simulink library "qcatlib"  (R2015a)
settings: Solver=ode45  SolverMode=SingleTasking  StartTime=0.0  StopTime=10.0  RelTol=1e-3
undefined symbols (not defined in the file or in its folder): dyn_ca_sl, qp_ca_sl
settings Model: CovSFcnEnable=off  ExtModeAutoUpdateStatusClock=off  Creator=ola  LastModifiedBy=David
settings DataIOCC: SignalLoggingSaveFormat=ModelDataLogs
settings OptimizationCC: BlockReduction=off  BooleanDataType=off  ExpressionDepthLimit=2147483647
settings DebuggingCC: SaveWithParameterizedLinksMsg=none  UnderspecifiedInitializationDetection=Classic  MergeDetectMultiDrivingBlocksExec=none  SignalResolutionControl=TryResolveAllWithWarning  MultiTaskDSMMsg=warning  MultiTaskCondExecSysMsg=none  StateNameClashWarn=warning  StrictBusMsg=None
settings HardwareCC: TargetUnknown=on

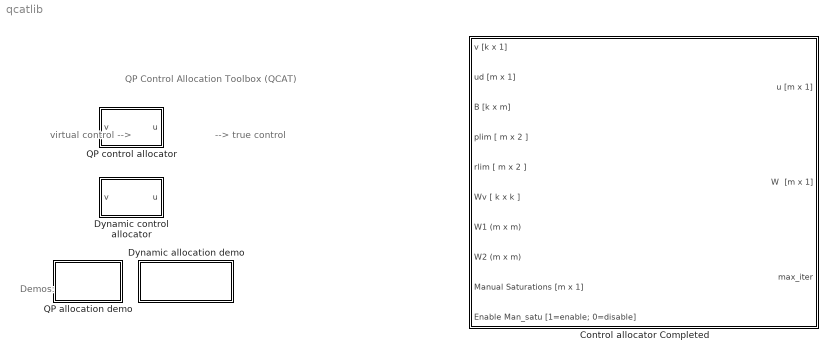
== system qcatlib ==
  note: virtual control -->
  note: --> true control
  note: QP Control Allocation Toolbox (QCAT)
  note: Demos:
  "Control allocator Completed " : Subsystem  TreatAsAtomicUnit=on  mask(Control allocator Completed){alg=WLS, CA_type=DYN, iter_max=100, gamma=1e6, k_B=3, m_B=7, T=0.01, tol=0}
      mask prompts: alg "Algorithm"; CA_type "CA type: Perform Dynamic CA?"; iter_max "Maximum number of iterations"; gamma "Weight of Control Error Cost (gamma) (If SLS, MLS or CGI:Include it in Wv)"; k_B "Number of rows B matrix"; m_B "Number of columns B Matrix"; T "Sample Time"; tol "Tolerance, tol"
      mask help:
      | Author: David Torres
      | Based on work of Ola Härkegård
      |
      | Given the virtual control command v:
      |  The control input u is computed using dynamic control allocation (see help dyn_ca_COMP).
      | OR
      |  The control input u is computed using l2-optimal control allocation (see help qp_ca_COMP).
      |
      | Type qcatdoc for more information.
      |
      | Note: CGI,FXP and IP do not manage saturations.
      mask Help: See the documentation for CA_COMP , dyn_ca_COMP or qp_ca_COMP.
      mask TypeOptions alg: SLS | WLS | WLSC | MLS | IP | CGI | FXP
      mask Callback alg:
      | val = get_param(gcb,'MaskValues');
      | switch lower(val{1})
      |  case {'sls','mls','cgi'}
      |   set_param(gcb,'MaskVisibilities',{'on','on','on','off','on','on','on','off'});
      |  case {'wls','wlsc','fxp'}
      |   set_param(gcb,'MaskVisibilities',{'on','on','on','on','on','on','on','off'});
      |  case {'ip'}
      |   set_param(gcb,'MaskVisibilities',{'on','on','on','on','on','on','on','on'});
      | end
      mask TypeOptions CA_type: DYN | QP
      mask Display:
      | fprintf('%s',upper(alg))
      | % %
      | % %
      | % % port_label('output', 1, 'u [m x 1]')
      | % % port_label('output', 2, 'W [m x 1]')
      | % % port_label('output', 3, 'iter max ')
      | % % port_label('input', 1, 'v [k x 1]')
      | % % port_label('input', 2, 'ud [m x 1]')
      | % % port_label('input', 3, 'B [k x m]')
      | % % port_label('input', 4, 'plim [m x 2]')
      | % % port_label('input', 5, 'rlim [m x 2]')
      | % % port_label('input', 6, 'Wv [k x k]')
      | % % port_label('input', 7, 'W1(u) [m x m]')
      | % % port_label('input', 8, 'W2 [m x m]')
      | % % port_label('input', 9, 'Manual Saturations [m x 1]')
  Dynamic allocation demo : Subsystem  mask{A=0}
      mask prompts: A "Needed for OpenSys to work from browser"
      settings: OpenFcn=open_system('dyn_alloc_demo')
      mask Display: disp('Dynamic control\nallocation')
  Dynamic control allocator : Subsystem  mask(Dynamic control allocator){B=[2 1], plim=[-1 1;-1 1], rlim=[-1 1;-1 1]*2, T=.1, Wv=1, W1=eye(2), W2=eye(2), S=[2 1]}
      mask prompts: B "Control effectiveness matrix, B"; plim "Position limits, plim"; rlim "Rate limits, rlim"; T "Sampling time, T"; Wv "Virtual control weighting matrix, Wv"; W1 "Control position weighting matrix, W1"; W2 "Control rate weighting matrix, W2"; S "Steady state distribution, S"
      mask help: Given the virtual control command v, the control input u is computed using dynamic control allocation (see help dyn_sim).
      mask Help: See the documentation for dyn_sim.
      mask Display: disp('Dynamic\nCA')
  QP allocation demo : Subsystem  mask{A=0}
      mask prompts: A "Needed for OpenSys to work from browser"
      settings: OpenFcn=open_system('qp_alloc_demo')
      mask Display: disp('QP control\nallocation')
  QP control allocator : Subsystem  AncestorBlock=qcatlib/Dynamic control allocator  mask(QP control allocator){B=[2 1], plim=[-1 1;-1 1], rlim=[-1 1;-1 1]*2, T=.1, Wv=1, Wu=eye(2), ud=[0 0]', alg=SLS, imax=100, gam=1e4, tol=1e-4}
      mask prompts: B "Control effectiveness matrix, B"; plim "Position limits, plim"; rlim "Rate limits, rlim"; T "Sampling time, T"; Wv "Virtual control weighting matrix, Wv"; Wu "Control weighting matrix, Wu"; ud "Desired control, ud"; alg "Algorithm"; imax "Max no. of iterations"; gam "Weight, gamma"; tol "Tolerance, tol"
      mask help: Given the virtual control command v, the control input u is computed using l2-optimal control allocation (see help qp_sim).
      mask Help: See the documentation for qp_sim.
      mask TypeOptions alg: SLS | WLS | WLSC | MLS | IP | CGI | FXP
      mask Callback alg:
      | val = get_param(gcb,'MaskValues');
      | switch lower(val{8})
      |  case {'sls','mls','cgi'}
      |   set_param(gcb,'MaskVisibilities',{'on','on','on','on','on','on','on','on','on','off','off'});
      |  case {'wls','wlsc','fxp'}
      |   set_param(gcb,'MaskVisibilities',{'on','on','on','on','on','on','on','on','on','on','off'});
      |  case {'ip'}
      |   set_param(gcb,'MaskVisibilities',{'on','on','on','on','off','off','on','on','on','on','on'});
      | end
      mask Display: fprintf('%s',upper(alg))

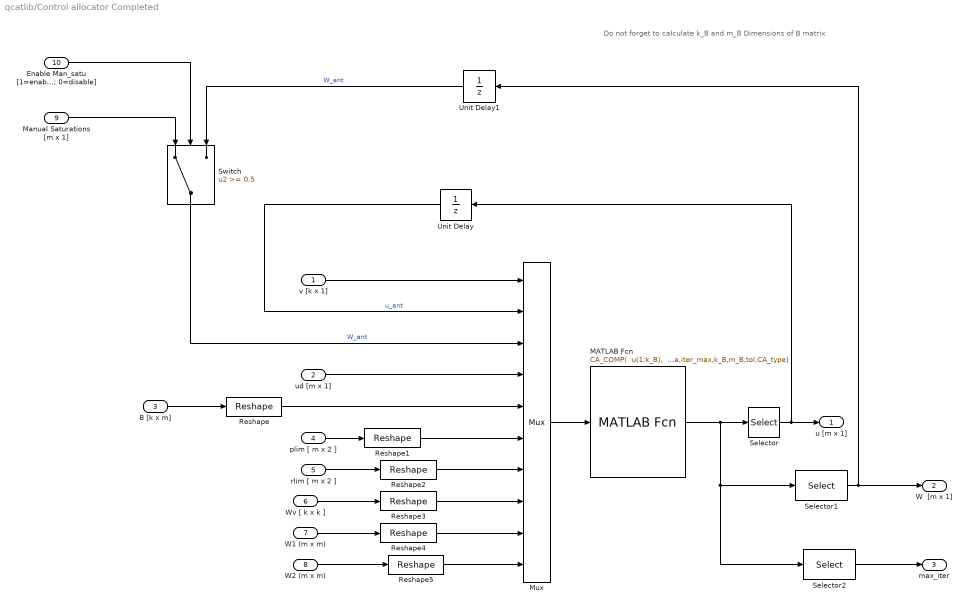
== system qcatlib/Control allocator Completed  ==
  note: Do not forget to calculate k_B and m_B Dimensions of B matrix
  v [k x 1] : Inport
  ud [m x 1] : Inport  Port=2
  B [k x m] : Inport  Port=3
  plim [ m x 2 ] : Inport  Port=4
  rlim [ m x 2 ] : Inport  Port=5
  Wv [ k x k ] : Inport  Port=6
  W1 (m x m) : Inport  Port=7
  W2 (m x m) : Inport  Port=8
  Manual Saturations [m x 1] : Inport  Port=9
  Enable Man_satu [1=enable; 0=disable] : Inport  Port=10
  MATLAB Fcn : MATLABFcn  MATLABFcn="CA_COMP(  u(1:k_B),  u(k_B+1:k_B+m_B),  u(k_B+m_B+1:k_B+2*m_B),  u(k_B+2*m_B+1:k_B+3*m_B),  u(k_B+3*m_B+1:k_B+3*m_B+m_B*k_B),  u(k_B+3*m_B+m_B*k_B+1:k_B+5*m_B+m_B*k_B),u(k_B+5*m_B+m_B*k_B+1:k_B+7*m_B+m_B*k_B),T,  u(k_B+7*m_B+m_B*k_B+1:k_B+7*m_B+m_B*k_B+k_B*k_B),  u(k_B+7*m_B+m_B*k_B+k_B*k_B+1:k_B+7*m_B+m_B*k_B+k_B*k_B+m_B*m_B),   u(k_B+7*m_B+m_B*k_B+k_B*k_B+m_B*m_B+1:k_B+7*m_B+m_B*k_B+k_B*k_B+2*m_B*m_B) ,   alg ,gamma,iter_max,k_B,m_B,tol,CA_type)"  OutputDimensions=m_B*2+1  SampleTime=T
  Mux : Mux  Inputs=10
  Reshape{,1..5} (6 alike) : Reshape  OutputDimensionality=Column vector (2-D)
  Selector : Selector  InputPortWidth=2*m_B+1  Indices=[1:m_B]
  Selector1 : Selector  InputPortWidth=m_B*2+1  Indices=[m_B+1:2*m_B]
  Selector2 : Selector  InputPortWidth=m_B*2+1  Indices=m_B*2+1
  Switch : Switch  Threshold=0.5  SampleTime=T
  Unit Delay : UnitDelay  InitialCondition=zeros(m_B,1)  SampleTime=T
  Unit Delay1 : UnitDelay  InitialCondition=zeros(m_B,1)  SampleTime=T
  u [m x 1] : Outport
  W  [m x 1] : Outport  Port=2
  max_iter : Outport  Port=3
  wires:
  MATLAB Fcn/1 -> Selector2/1, Selector1/1, Selector/1
  v [k x 1]/1 -> Mux/1
  Mux/1 -> MATLAB Fcn/1
  Unit Delay/1 -> Mux/2  "u_ant"
  B [k x m]/1 -> Reshape/1
  plim [ m x 2 ]/1 -> Reshape1/1
  rlim [ m x 2 ]/1 -> Reshape2/1
  Wv [ k x k ]/1 -> Reshape3/1
  W1 (m x m)/1 -> Reshape4/1
  W2 (m x m)/1 -> Reshape5/1
  Reshape/1 -> Mux/5
  ud [m x 1]/1 -> Mux/4
  Selector1/1 -> Unit Delay1/1, W  [m x 1]/1
  Switch/1 -> Mux/3  "W_ant"
  Selector/1 -> u [m x 1]/1, Unit Delay/1
  Reshape1/1 -> Mux/6
  Reshape2/1 -> Mux/7
  Reshape3/1 -> Mux/8
  Reshape4/1 -> Mux/9
  Reshape5/1 -> Mux/10
  Selector2/1 -> max_iter/1
  Unit Delay1/1 -> Switch/3  "W_ant"
  Manual Saturations [m x 1]/1 -> Switch/1
  Enable Man_satu [1=enable; 0=disable]/1 -> Switch/2

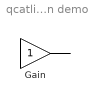
== system qcatlib/Dynamic allocation demo ==
  Gain : Gain  SaturateOnIntegerOverflow=on  OutDataTypeStr=Inherit: Same as input  ParamDataTypeStr=Inherit: Same as input
  wires:
  ? -> Gain/1
  Gain/1 -> ?

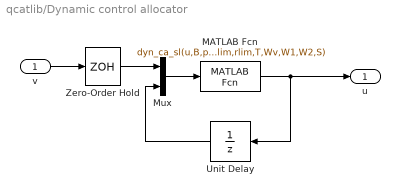
== system qcatlib/Dynamic control allocator ==
  v : Inport
  MATLAB Fcn : MATLABFcn  MATLABFcn=dyn_ca_sl(u,B,plim,rlim,T,Wv,W1,W2,S)  OutputDimensions=size(B,2)
  Mux : Mux  Inputs=2
  Unit Delay : UnitDelay  SampleTime=T
  Zero-Order Hold : ZeroOrderHold  SampleTime=T
  u : Outport
  wires:
  Unit Delay/1 -> Mux/2
  Mux/1 -> MATLAB Fcn/1
  Zero-Order Hold/1 -> Mux/1
  MATLAB Fcn/1 -> Unit Delay/1, u/1
  v/1 -> Zero-Order Hold/1

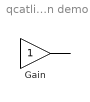
== system qcatlib/QP allocation demo ==
  Gain : Gain  SaturateOnIntegerOverflow=on  OutDataTypeStr=Inherit: Same as input  ParamDataTypeStr=Inherit: Same as input
  wires:
  ? -> Gain/1
  Gain/1 -> ?

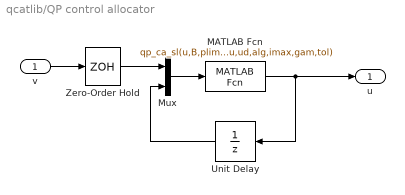
== system qcatlib/QP control allocator ==
  v : Inport
  MATLAB Fcn : MATLABFcn  MATLABFcn=qp_ca_sl(u,B,plim,rlim,T,Wv,Wu,ud,alg,imax,gam,tol)  OutputDimensions=size(B,2)
  Mux : Mux  Inputs=2
  Unit Delay : UnitDelay  SampleTime=T
  Zero-Order Hold : ZeroOrderHold  SampleTime=T
  u : Outport
  wires:
  v/1 -> Zero-Order Hold/1
  Unit Delay/1 -> Mux/2
  Mux/1 -> MATLAB Fcn/1
  Zero-Order Hold/1 -> Mux/1
  MATLAB Fcn/1 -> u/1, Unit Delay/1
